simulink library "libbestfx"  (R2018b)
settings: Solver=VariableStepAuto  StartTime=0.0  StopTime=10.0  RelTol=1e-3
undefined symbols (not defined in the file or in its folder): R, S, VariantTypeR, VariantTypeS
libraries: simulink x25, $bdroot x14
(part 2 of 2)

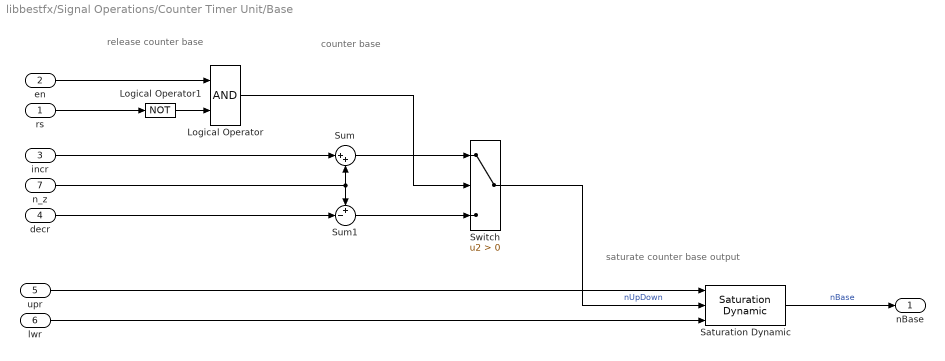
== system libbestfx/Signal Operations/Counter Timer Unit/Base ==
  note: counter base
  note: release counter base
  note: saturate counter base output
  rs : Inport
  en : Inport  Port=2
  incr : Inport  Port=3
  decr : Inport  Port=4
  upr : Inport  Port=5
  lwr : Inport  Port=6
  n_z : Inport  Port=7
  Logical Operator : Logic  AllPortsSameDT=off  OutDataTypeStr=boolean
  Logical Operator1 : Logic  Operator=NOT  AllPortsSameDT=off  OutDataTypeStr=boolean
  Saturation Dynamic : simulink/Discontinuities/Saturation Dynamic  OutMin=[]  OutMax=[]  OutDataTypeStr=Inherit: Same as second input  OutDataType=fixdt(1, 16)  OutScaling=2^-10  DoSatur=off
  Sum : Sum  Inputs=|++  SaturateOnIntegerOverflow=on
      settings: AttributesFormatString=IOP: on
  Sum1 : Sum  Inputs=+-|  SaturateOnIntegerOverflow=on
      settings: AttributesFormatString=IOP: on
  Switch : Switch  Criteria=u2 > Threshold
      settings: AttributesFormatString=%<Criteria> \n Threshold: %<Threshold>
  nBase : Outport
  wires:
  en/1 -> Logical Operator/1
  rs/1 -> Logical Operator1/1
  decr/1 -> Sum1/2
  Logical Operator/1 -> Switch/2
  Sum/1 -> Switch/1
  n_z/1 -> Sum/2, Sum1/1
  incr/1 -> Sum/1
  Sum1/1 -> Switch/3
  Logical Operator1/1 -> Logical Operator/2
  Switch/1 -> Saturation Dynamic/2  "nUpDown"
  Saturation Dynamic/1 -> nBase/1  "nBase"
  lwr/1 -> Saturation Dynamic/3
  upr/1 -> Saturation Dynamic/1

== system libbestfx/Signal Operations/Counter Timer Unit/VariantReset ==
  note: 1) Add Subsystem or Model blocks as valid variant choices.
      | 2) You cannot connect blocks at this level. At simulation, connectivity is automatically
      | determined, based on the active variant and port name matching.
  u : Inport
  st : Inport  Port=2
  FreeRunning : Subsystem  VariantControl=VariantResetFreeRunning
  PassThrough : Subsystem  VariantControl=VariantResetPassThrough
  n : Outport

== system libbestfx/Signal Operations/Counter Timer Unit/VariantState ==
  note: 1) Add Subsystem or Model blocks as valid variant choices.
      | 2) You cannot connect blocks at this level. At simulation, connectivity is automatically
      | determined, based on the active variant and port name matching.
  n : Inport
  upr : Inport  Port=2
  lwr : Inport  Port=3
  Bidirectional : Subsystem  VariantControl=VariantStateBidirectional
  Level : Subsystem  VariantControl=VariantStateLevel
  st : Outport

== system libbestfx/Signal Operations/Counter Timer Unit/VariantType ==
  note: 1) Add Subsystem or Model blocks as valid variant choices.
      | 2) You cannot connect blocks at this level. At simulation, connectivity is automatically
      | determined, based on the active variant and port name matching.
  rs : Inport
  u : Inport  Port=2
  x0 : Inport  Port=3
  Counter : Subsystem  VariantControl=VariantTypeCounter
  Timer : Subsystem  VariantControl=VariantTypeTimer
  n : Outport
  y : Outport  Port=2

== system libbestfx/Signal Operations/Counter Timer Unit/Virtual Unit Delay ==
  u : Inport
  y : Outport
  wires:
  u/1 -> y/1

== system libbestfx/Signal Operations/Counter Timer Unit/Virtual Unit Delay1 ==
  u : Inport
  y : Outport
  wires:
  u/1 -> y/1

== system libbestfx/Signal Operations/Debounce Unit/Count ==
  en : Inport
  n : Inport  Port=2
  Constant1 : Constant  OutDataTypeStr=Inherit: Inherit via back propagation
  Relational Operator : RelationalOperator  Operator=<  OutDataTypeStr=boolean  RndMeth=Simplest
  Sum : Sum  Inputs=++|
  Switch : Switch  Criteria=u2 > Threshold
      settings: AttributesFormatString=%<Criteria> \n Threshold: %<Threshold>
  Unit Delay : UnitDelay  InitialCondition=1  SampleTime=-1
      settings: AttributesFormatString=IC=1
  rs : Outport
  wires:
  n/1 -> Relational Operator/1
  Relational Operator/1 -> rs/1
  Constant1/1 -> Switch/3, Sum/1
  Sum/1 -> Switch/1
  Unit Delay/1 -> Relational Operator/2, Sum/2  "cntr"
  en/1 -> Switch/2
  Switch/1 -> Unit Delay/1

== system libbestfx/Signal Operations/Debounce Unit/VariantControl ==
  "u " : Inport
  NoReset : Subsystem  VariantControl=VariantControlNoReset
  Normal : Subsystem  VariantControl=VariantControlNormal
  Swapped : Subsystem  VariantControl=VariantControlSwapped
  set : Outport
  rs : Outport  Port=2

== system libbestfx/Signal Operations/Debounce Unit/VariantDebounce ==
  "u " : Inport
  "tf " : Inport  Port=2
  CaptureHold : Subsystem  VariantControl=VariantDebounceCaptureHold
  PassThrough : Subsystem  VariantControl=VariantDebouncePassThrough
  ZeroHold : Subsystem  VariantControl=VariantDebounceZeroHold
  " y" : Outport

== system libbestfx/Signal Operations/Debounce Unit/Virtual Unit Delay ==
  u : Inport
  y : Outport
  wires:
  u/1 -> y/1

== system libbestfx/Signal Operations/Flip-Flop/VariantType ==
  "u " : Inport
  R-S : Subsystem  VariantControl=VariantTypeR-S
  S-R : Subsystem  VariantControl=VariantTypeS-R
  " y" : Outport

== system libbestfx/Signal Operations/Pulse Divider/Edge Counter ==
  edge : Inport
  k : Inport  Port=2
  Constant : Constant  OutDataTypeStr=Inherit: Inherit via back propagation
  Data Type Duplicate : DataTypeDuplicate
  Relational Operator : RelationalOperator  Operator=<=  OutDataTypeStr=boolean  RndMeth=Simplest
  Sum : Sum  Inputs=++|
  Switch : Switch  Criteria=u2 > Threshold
      settings: AttributesFormatString=%<Criteria> \n Threshold: %<Threshold>
  Unit Delay : UnitDelay  SampleTime=-1
  cntr : Outport
  wires:
  k/1 -> Data Type Duplicate/1, Relational Operator/1
  Unit Delay/1 -> Relational Operator/2, Switch/3
  edge/1 -> Sum/1
  Switch/1 -> Sum/2
  Relational Operator/1 -> Switch/2
  Sum/1 -> Unit Delay/1, cntr/1  "cntr"
  Constant/1 -> Data Type Duplicate/2, Switch/1

== system libbestfx/Signal Operations/Pulse Divider/Toggle ==
  u : Inport
  NOT : Logic  Operator=NOT  AllPortsSameDT=off  OutDataTypeStr=boolean
  Switch : Switch  Criteria=u2 > Threshold
      settings: AttributesFormatString=%<Criteria> \n Threshold: %<Threshold>
  Unit Delay : UnitDelay  InitialCondition=1  SampleTime=-1
      settings: AttributesFormatString=IC=1
  y : Outport
  wires:
  NOT/1 -> Switch/1
  Switch/1 -> Unit Delay/1, y/1
  u/1 -> Switch/2
  Unit Delay/1 -> NOT/1, Switch/3

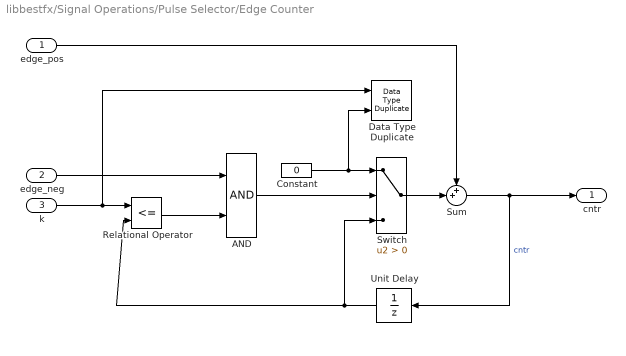
== system libbestfx/Signal Operations/Pulse Selector/Edge Counter ==
  edge_pos : Inport
  edge_neg : Inport  Port=2
  k : Inport  Port=3
  AND : Logic  AllPortsSameDT=off  OutDataTypeStr=boolean
  Constant : Constant  Value=0  OutDataTypeStr=Inherit: Inherit via back propagation
  Data Type Duplicate : DataTypeDuplicate
  Relational Operator : RelationalOperator  Operator=<=  OutDataTypeStr=boolean  RndMeth=Simplest
  Sum : Sum  Inputs=++|
  Switch : Switch  Criteria=u2 > Threshold
      settings: AttributesFormatString=%<Criteria> \n Threshold: %<Threshold>
  Unit Delay : UnitDelay  SampleTime=-1
  cntr : Outport
  wires:
  AND/1 -> Switch/2
  edge_neg/1 -> AND/1
  Relational Operator/1 -> AND/2
  edge_pos/1 -> Sum/1
  k/1 -> Relational Operator/1, Data Type Duplicate/1
  Unit Delay/1 -> Relational Operator/2, Switch/3
  Switch/1 -> Sum/2
  Sum/1 -> Unit Delay/1, cntr/1  "cntr"
  Constant/1 -> Data Type Duplicate/2, Switch/1

== system libbestfx/Signal Processing/Discrete Filter/VariantType ==
  "T " : Inport
  "u " : Inport  Port=2
  Highpass : Subsystem  VariantControl=VariantTypeHighpass
  Lowpass : Subsystem  VariantControl=VariantTypeLowpass
  " y" : Outport

== system libbestfx/Signal Verification/Validate/VariantRange ==
  note: 1) Add Subsystem or Model blocks as valid variant choices.
      | 2) You cannot connect blocks at this level. At simulation, connectivity is automatically
      | determined, based on the active variant and port name matching.
  u : Inport
  lwr : Inport  Port=2
  upr : Inport  Port=3
  Above : Subsystem  VariantControl=VariantRangeAbove
  Below : Subsystem  VariantControl=VariantRangeBelow
  Inside : Subsystem  VariantControl=VariantRangeInside
  None : Subsystem  VariantControl=VariantRangeNone
  state : Outport

== system libbestfx/Signal Verification/Validate/VariantType ==
  note: 1) Add Subsystem or Model blocks as valid variant choices.
      | 2) You cannot connect blocks at this level. At simulation, connectivity is automatically
      | determined, based on the active variant and port name matching.
  state : Inport
  u : Inport  Port=2
  PassThrough : Subsystem  VariantControl=VariantTypePassThrough
  Stuck : Subsystem  VariantControl=VariantTypeStuck
  valid : Outport

== system libbestfx/Signal Attributes/Data Pack/VariantSpecifier/PassThrough ==
  u : Inport
  y : Outport
  wires:
  u/1 -> y/1

== system libbestfx/Signal Attributes/Data Pack/VariantSpecifier/Signed ==
  u : Inport
  Saturation : Saturate  UpperLimit=2^(Length-1)-1  LowerLimit=-2^(Length-1)  OutDataTypeStr=OutputDataType
      settings: AttributesFormatString=[-2^(Length-1) .. 2^(Length-1)-1]
  y : Outport
  wires:
  u/1 -> Saturation/1
  Saturation/1 -> y/1

== system libbestfx/Signal Attributes/Data Pack/VariantSpecifier/Unsigned ==
  u : Inport
  Saturation : Saturate  UpperLimit=2^Length-1  LowerLimit=0  OutDataTypeStr=OutputDataType
      settings: AttributesFormatString=[0 .. 2^Length-1]
  y : Outport
  wires:
  Saturation/1 -> y/1
  u/1 -> Saturation/1

== system libbestfx/Signal Attributes/Data Unpack/VariantSpecifier/PassThrough ==
  u : Inport
  y : Outport
  wires:
  u/1 -> y/1

== system libbestfx/Signal Attributes/Data Unpack/VariantSpecifier/Signed ==
  u : Inport
  Saturation : Saturate  UpperLimit=2^(Length-1)-1  LowerLimit=-2^(Length-1)
      settings: AttributesFormatString=[-2^(Length-1) .. 2^(Length-1)-1]
  y : Outport
  wires:
  u/1 -> Saturation/1
  Saturation/1 -> y/1

== system libbestfx/Signal Attributes/Data Unpack/VariantSpecifier/Unsigned ==
  u : Inport
  Saturation : Saturate  UpperLimit=2^Length-1  LowerLimit=0
      settings: AttributesFormatString=[0 .. 2^Length-1]
  y : Outport
  wires:
  Saturation/1 -> y/1
  u/1 -> Saturation/1

== system libbestfx/Signal Operations/Counter Timer Unit/VariantReset/FreeRunning ==
  u : Inport
  st : Inport  Port=2
  Logical Operator : Logic  Operator=OR  AllPortsSameDT=off  OutDataTypeStr=boolean
  Unit Delay : UnitDelay  SampleTime=-1
  n : Outport
  wires:
  Logical Operator/1 -> n/1
  u/1 -> Logical Operator/1
  Unit Delay/1 -> Logical Operator/2
  st/1 -> Unit Delay/1

== system libbestfx/Signal Operations/Counter Timer Unit/VariantReset/PassThrough ==
  u : Inport
  n : Outport
  wires:
  u/1 -> n/1

== system libbestfx/Signal Operations/Counter Timer Unit/VariantState/Bidirectional ==
  n : Inport
  upr : Inport  Port=2
  lwr : Inport  Port=3
  Flip-Flop : $bdroot/Signal Operations/Flip-Flop  BlockSubtypeVariant=Bistable R-S  StateSourcePort=on  NegatedStateSourcePort=off  InitialCondition=false
      settings: AttributesFormatString=%<BlockSubtypeVariant>
  Relational Operator : RelationalOperator  Operator=<=  OutDataTypeStr=boolean  RndMeth=Nearest
  Relational Operator1 : RelationalOperator  Operator=<=  OutDataTypeStr=boolean  RndMeth=Nearest
  st : Outport
  wires:
  upr/1 -> Relational Operator/1
  n/1 -> Relational Operator1/1, Relational Operator/2
  lwr/1 -> Relational Operator1/2
  Relational Operator/1 -> Flip-Flop/1
  Relational Operator1/1 -> Flip-Flop/2
  Flip-Flop/1 -> st/1

== system libbestfx/Signal Operations/Counter Timer Unit/VariantState/Level ==
  n : Inport
  upr : Inport  Port=2
  Relational Operator : RelationalOperator  Operator=<=  OutDataTypeStr=boolean  RndMeth=Nearest
  st : Outport
  wires:
  Relational Operator/1 -> st/1
  upr/1 -> Relational Operator/1
  n/1 -> Relational Operator/2

== system libbestfx/Signal Operations/Counter Timer Unit/VariantType/Counter ==
  note: Reset Mode Behavior:
      |
      | [ ] None No reset
      | [ ] Rising Reset on a rising edge
      | [ ] Falling Reset on a falling edge
      | [ ] Either Reset on either a rising or falling edge
      | [ ] Level Reset in either of these cases:
      | - When the reset signal is nonzero at the current time step
      | - When the reset signal value changes from nonzero at the previous time step to zero at the current time step
      | [X] Level hold
      | - Reset when the reset signal is nonzero at the current time step
  rs : Inport
  u : Inport  Port=2
  x0 : Inport  Port=3
  Counter State : Delay  DelayLength=1  InitialConditionSource=Input port  ExternalReset=Level hold
      settings: InputPortMap=u0,r5,p4
  n : Outport
  y : Outport  Port=2
  wires:
  Counter State/1 -> y/1
  u/1 -> Counter State/1, n/1
  x0/1 -> Counter State/3
  rs/1 -> Counter State/2

== system libbestfx/Signal Operations/Counter Timer Unit/VariantType/Timer ==
  note: Reset Mode Behavior:
      |
      | [ ] None No reset
      | [ ] Rising Reset on a rising edge
      | [ ] Falling Reset on a falling edge
      | [ ] Either Reset on either a rising or falling edge
      | [ ] Level Reset in either of these cases:
      | - When the reset signal is nonzero at the current time step
      | - When the reset signal value changes from nonzero at the previous time step to zero at the current time step
      | [X] Level hold
      | - Reset when the reset signal is nonzero at the current time step
  rs : Inport
  u : Inport  Port=2
  x0 : Inport  Port=3
  Timer State : Delay  DelayLength=1  InitialConditionSource=Input port  ExternalReset=Level hold
      settings: InputPortMap=u0,r5,p4
  n : Outport
  y : Outport  Port=2
  wires:
  u/1 -> Timer State/1
  Timer State/1 -> n/1, y/1
  x0/1 -> Timer State/3
  rs/1 -> Timer State/2

== system libbestfx/Signal Operations/Debounce Unit/VariantControl/NoReset ==
  "u " : Inport
  False : Constant  Value=false  OutDataTypeStr=Inherit: Inherit via back propagation
  Relational Operator : RelationalOperator  Operator=>  OutDataTypeStr=boolean  ZeroCross=off  RndMeth=Nearest
  UD : UnitDelay  Description=Store in Global RAM  DisableCoverage=on  InitialCondition=0.0  SampleTime=-1
  set : Outport
  rs : Outport  Port=2
  wires:
  "u "/1 -> UD/1, Relational Operator/1  "u(k)"
  UD/1 -> Relational Operator/2  "u(k-1)"
  Relational Operator/1 -> set/1  "U>Uz"
  False/1 -> rs/1

== system libbestfx/Signal Operations/Debounce Unit/VariantControl/Normal ==
  "u " : Inport
  Relational Operator : RelationalOperator  Operator=>  OutDataTypeStr=boolean  ZeroCross=off  RndMeth=Nearest
  Relational Operator1 : RelationalOperator  Operator=<  OutDataTypeStr=boolean  ZeroCross=off  RndMeth=Nearest
  UD : UnitDelay  Description=Store in Global RAM  DisableCoverage=on  InitialCondition=0.0  SampleTime=-1
  set : Outport
  rs : Outport  Port=2
  wires:
  Relational Operator/1 -> set/1  "U>Uz"
  UD/1 -> Relational Operator/2, Relational Operator1/2  "u(k-1)"
  "u "/1 -> Relational Operator/1, Relational Operator1/1, UD/1  "u(k)"
  Relational Operator1/1 -> rs/1  "U<Uz"

== system libbestfx/Signal Operations/Debounce Unit/VariantControl/Swapped ==
  "u " : Inport
  Relational Operator : RelationalOperator  Operator=>  OutDataTypeStr=boolean  ZeroCross=off  RndMeth=Nearest
  Relational Operator1 : RelationalOperator  Operator=<  OutDataTypeStr=boolean  ZeroCross=off  RndMeth=Nearest
  UD : UnitDelay  Description=Store in Global RAM  DisableCoverage=on  InitialCondition=0.0  SampleTime=-1
  set : Outport
  rs : Outport  Port=2
  wires:
  Relational Operator1/1 -> set/1  "U<Uz"
  "u "/1 -> UD/1, Relational Operator1/1, Relational Operator/1  "u(k)"
  UD/1 -> Relational Operator1/2, Relational Operator/2  "u(k-1)"
  Relational Operator/1 -> rs/1  "U>Uz"

== system libbestfx/Signal Operations/Debounce Unit/VariantDebounce/CaptureHold ==
  u : Inport
  "tf " : Inport  Port=2
  Max : MinMax  Function=max  Inputs=2
  Switch1 : Switch  Criteria=u2 > Threshold
      settings: AttributesFormatString=%<Criteria> \n Threshold: %<Threshold>
  Unit Delay1 : UnitDelay  SampleTime=-1
  y : Outport
  wires:
  "tf "/1 -> Switch1/2
  Switch1/1 -> y/1, Unit Delay1/1
  u/1 -> Max/1, Switch1/3
  Max/1 -> Switch1/1
  Unit Delay1/1 -> Max/2

== system libbestfx/Signal Operations/Debounce Unit/VariantDebounce/PassThrough ==
  u : Inport
  y : Outport
  wires:
  u/1 -> y/1

== system libbestfx/Signal Operations/Debounce Unit/VariantDebounce/ZeroHold ==
  u : Inport
  "tf " : Inport  Port=2
  Switch To Zero : $bdroot/Signal Operations/Switch To Zero
  y : Outport
  wires:
  Switch To Zero/1 -> y/1
  u/1 -> Switch To Zero/1
  "tf "/1 -> Switch To Zero/2

== system libbestfx/Signal Operations/Flip-Flop/VariantType/R-S ==
  "u " : Inport
  Logic : CombinatorialLogic  TruthTable=[0 1;1 0;0 1;0 1;1 0;1 0;0 1;0 1]
  " y" : Outport
  wires:
  Logic/1 -> " y"/1
  "u "/1 -> Logic/1

== system libbestfx/Signal Operations/Flip-Flop/VariantType/S-R ==
  "u " : Inport
  Logic : CombinatorialLogic  TruthTable=[0 1;1 0;0 1;0 1;1 0;1 0;1 0;1 0]
  " y" : Outport
  wires:
  "u "/1 -> Logic/1
  Logic/1 -> " y"/1

== system libbestfx/Signal Processing/Discrete Filter/VariantType/Highpass ==
  u : Inport
  Sum3 : Sum  Inputs=|+-
  Unit Delay2 : UnitDelay  SampleTime=-1
  y : Outport
  wires:
  Sum3/1 -> y/1
  u/1 -> Sum3/1, Unit Delay2/1
  Unit Delay2/1 -> Sum3/2

== system libbestfx/Signal Processing/Discrete Filter/VariantType/Lowpass ==
  T : Inport
  u : Inport  Port=2
  Constant2 : Constant  OutDataTypeStr=Inherit: Inherit via back propagation
  Data Type Duplicate : DataTypeDuplicate
  Product2 : Product
  Sum : Sum  Inputs=-+|  OutDataTypeStr=Inherit: Same as first input
  y : Outport
  wires:
  Sum/1 -> Product2/1
  Product2/1 -> y/1
  Constant2/1 -> Sum/2, Data Type Duplicate/2
  T/1 -> Sum/1
  u/1 -> Product2/2, Data Type Duplicate/1

== system libbestfx/Signal Verification/Validate/VariantRange/Above ==
  u : Inport
  upr : Inport  Port=2
  Relational Operator1 : RelationalOperator  Operator=<=  OutDataTypeStr=boolean  RndMeth=Simplest
  state : Outport
  wires:
  Relational Operator1/1 -> state/1
  upr/1 -> Relational Operator1/1
  u/1 -> Relational Operator1/2

== system libbestfx/Signal Verification/Validate/VariantRange/Below ==
  u : Inport
  lwr : Inport  Port=2
  Relational Operator1 : RelationalOperator  Operator=<=  OutDataTypeStr=boolean  RndMeth=Simplest
  state : Outport
  wires:
  u/1 -> Relational Operator1/1
  Relational Operator1/1 -> state/1
  lwr/1 -> Relational Operator1/2

== system libbestfx/Signal Verification/Validate/VariantRange/Inside ==
  u : Inport
  lwr : Inport  Port=2
  upr : Inport  Port=3
  Logical Operator : Logic  AllPortsSameDT=off  OutDataTypeStr=boolean
  Relational Operator : RelationalOperator  Operator=<=  OutDataTypeStr=boolean  RndMeth=Simplest
  Relational Operator1 : RelationalOperator  Operator=<=  OutDataTypeStr=boolean  RndMeth=Simplest
  state : Outport
  wires:
  Relational Operator/1 -> Logical Operator/1
  Relational Operator1/1 -> Logical Operator/2
  u/1 -> Relational Operator1/1, Relational Operator/2
  Logical Operator/1 -> state/1
  lwr/1 -> Relational Operator/1
  upr/1 -> Relational Operator1/2

== system libbestfx/Signal Verification/Validate/VariantRange/None ==
  Constant : Constant  Value=true
  state : Outport
  wires:
  Constant/1 -> state/1

== system libbestfx/Signal Verification/Validate/VariantType/PassThrough ==
  state : Inport
  valid : Outport
  wires:
  state/1 -> valid/1

== system libbestfx/Signal Verification/Validate/VariantType/Stuck ==
  state : Inport
  u : Inport  Port=2
  Detect Change : simulink/Logic and Bit Operations/Detect Change  vinit=0  OutDataTypeStr=boolean
  Logical Operator2 : Logic  Operator=NOT  Inputs=NOT  AllPortsSameDT=off  OutDataTypeStr=boolean
  NAND : Logic  Operator=NAND  AllPortsSameDT=off  OutDataTypeStr=boolean
  valid : Outport
  wires:
  u/1 -> Detect Change/1
  Detect Change/1 -> Logical Operator2/1
  Logical Operator2/1 -> NAND/2  "stuck"
  state/1 -> NAND/1
  NAND/1 -> valid/1
